simulink model "ex1_model"  (R2022a)
settings: Solver=VariableStepAuto  StartTime=0.0  StopTime=10.0  RelTol=1e-3
values from neighbouring files (symbols this model uses):
  B = 4    [ex1_para.m]    (also in ex2_plot.m = 25)
  K = 16    [ex1_para.m]
  M = 2    [ex1_para.m]
settings Model: Creator=du3781xx  LastModifiedBy=du3781xx

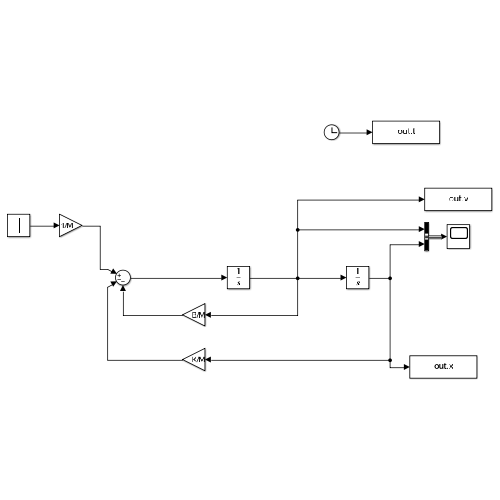
[thumbnail: Simulink's stored preview of the top-level diagram]
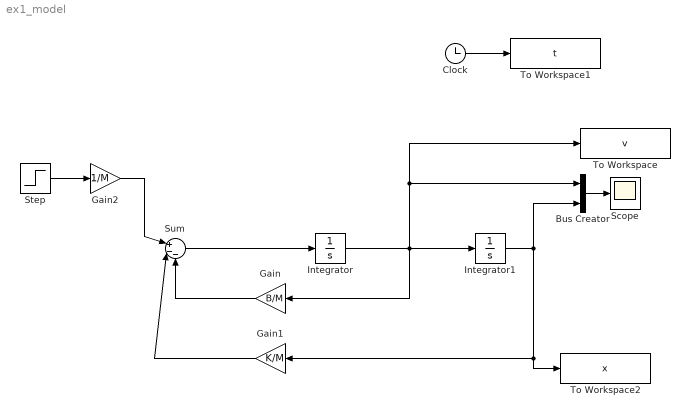
== system ex1_model ==
  Bus Creator : BusCreator  Inputs=2
  Clock : Clock
  Gain : Gain  Gain=B/M
  Gain1 : Gain  Gain=K/M
  Gain2 : Gain  Gain=1/M
  Integrator : Integrator
  Integrator1 : Integrator
  Scope : Scope
  Step : Step  After=8  SampleTime=0
  Sum : Sum  Inputs=|+--
  To Workspace : ToWorkspace  VariableName=v  SaveFormat=Timeseries  SampleTime=-1
  To Workspace1 : ToWorkspace  VariableName=t  SaveFormat=Timeseries  SampleTime=-1
  To Workspace2 : ToWorkspace  VariableName=x  SaveFormat=Timeseries  SampleTime=-1
  wires:
  Step/1 -> Gain2/1
  Gain2/1 -> Sum/1
  Sum/1 -> Integrator/1
  Integrator/1 -> Integrator1/1, Gain/1, To Workspace/1, Bus Creator/1
  Gain/1 -> Sum/3
  Gain1/1 -> Sum/2
  Clock/1 -> To Workspace1/1
  Integrator1/1 -> Bus Creator/2, Gain1/1, To Workspace2/1
  Bus Creator/1 -> Scope/1
